simulink model "JacobiansTest"  (Simulink 7.9)
settings: Solver=ode45  StartTime=0.0  StopTime=inf  RelTol=1e-3
libraries: WBCLibrary x5, dspmtrx3 x2, simulink x1
settings Model: Creator=jorhabib  LastModifiedBy=jorhabib
settings SFSimCC: SimParseCustomCode=off
settings CodeAppCC: CustomSymbolStrType=$N$R$M_T
settings GRTTargetCC: CodeReplacementLibrary=C89/C90 (ANSI)

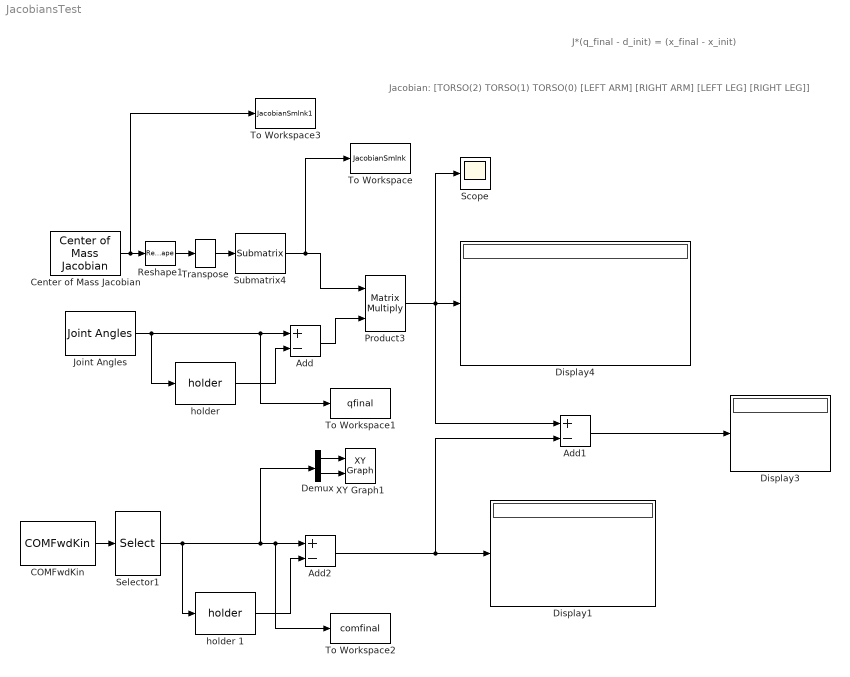
== system JacobiansTest ==
  note: Jacobian: [TORSO(2) TORSO(1) TORSO(0) [LEFT ARM] [RIGHT ARM] [LEFT LEG] [RIGHT LEG]]
  note: J*(q_final - d_init) = (x_final - x_init)
  Add : Sum  Inputs=+-
  Add1 : Sum  Inputs=+-
  Add2 : Sum  Inputs=+-
  "COMFwdKin " : WBCLibrary/wholeBodyModel/Forward Kinematics/COMFwdKin   robotName=robotName  localName=localName
  Center of Mass Jacobian : WBCLibrary/wholeBodyModel/Jacobians/Center of Mass Jacobian  robotName=robotName  localName=localName
  Demux : Demux  Outputs=2
  Display1 : Display
  Display3 : Display
  Display4 : Display
  Joint Angles : WBCLibrary/wholeBodyStates/Joint Angles  robotName=robotName  localName=localName
  Product3 : Product  Multiplication=Matrix(*)  RndMeth=Zero
  Reshape1 : Reshape  OutputDimensionality=Customize  OutputDimensions=[31,6]
  Scope : Scope
      settings: ShowLegends=on  TimeRange=100  YMin=-0.005  YMax=0.04
  Selector1 : Selector  IndexMode=Zero-based  InputPortWidth=7  Indices=[0:1]
  Submatrix4 : dspmtrx3/Submatrix  RowSpan=Range of rows  RowStartMode=First  RowStartIndex=1  RowEndMode=Index  RowEndIndex=2  ColSpan=Range of columns  ColStartMode=Index  ColStartIndex=7  ColEndMode=Last  ColEndIndex=6
  To Workspace : ToWorkspace  VariableName=JacobianSmlnk  SampleTime=-1
  To Workspace1 : ToWorkspace  VariableName=qfinal  SampleTime=-1
  To Workspace2 : ToWorkspace  VariableName=comfinal  SampleTime=-1
  To Workspace3 : ToWorkspace  VariableName=JacobianSmlnk1  SampleTime=-1
  Transpose : dspmtrx3/Transpose  Hermitian=off  overflowFlag=off
  XY Graph1 : simulink/Sinks/XY Graph  xmin=0.0125  xmax=0.035  ymin=-0.2  ymax=-0.1  st=-1
  "holder " : WBCLibrary/Utilities/holder 
  holder 1 : WBCLibrary/Utilities/holder 
  wires:
  Center of Mass Jacobian/1 -> Reshape1/1, To Workspace3/1
  Reshape1/1 -> Transpose/1
  Submatrix4/1 -> Product3/1, To Workspace/1
  "COMFwdKin "/1 -> Selector1/1
  Selector1/1 -> holder 1/1, Demux/1, Add2/1, To Workspace2/1
  Product3/1 -> Display4/1, Add1/1, Scope/1
  Joint Angles/1 -> "holder "/1, Add/1, To Workspace1/1
  Add/1 -> Product3/2
  "holder "/1 -> Add/2
  Add1/1 -> Display3/1
  holder 1/1 -> Add2/2
  Add2/1 -> Display1/1, Add1/2
  Demux/1 -> XY Graph1/1
  Demux/2 -> XY Graph1/2
  Transpose/1 -> Submatrix4/1
